simulink model "Acquisition_from_autosave"  (R2017a)
settings: Solver=VariableStepAuto  StartTime=0.0  StopTime=0.5  RelTol=1e-3
undefined symbols (not defined in the file): magnitude, Radix
libraries: simulink x34, commfilt2 x30, dspswit3 x12, dspmtrx3 x12, dspxfrm3 x3, simulink_extras x2, dspbuff3 x1
(part 1 of 4)
settings Model: Creator=Alam  LastModifiedBy=Alam
settings SolverCC: AutoInsertRateTranBlk=on
settings DataIOCC: LimitDataPoints=on  SaveOutput=off  SignalLogging=off  SaveTime=off
settings OptimizationCC: LifeSpan=inf
settings DebuggingCC: AlgebraicLoopMsg=none  SingleTaskRateTransMsg=error  AllowSymbolicDim=off  SFUnexpectedBacktrackingDiag=warning  SFNoUnconditionalDefaultTransitionDiag=warning  SFExecutionAtInitializationDiag=none
settings GRTTargetCC: TargetLangStandard=C89/C90 (ANSI)  GeneratePreprocessorConditionals=Disable all

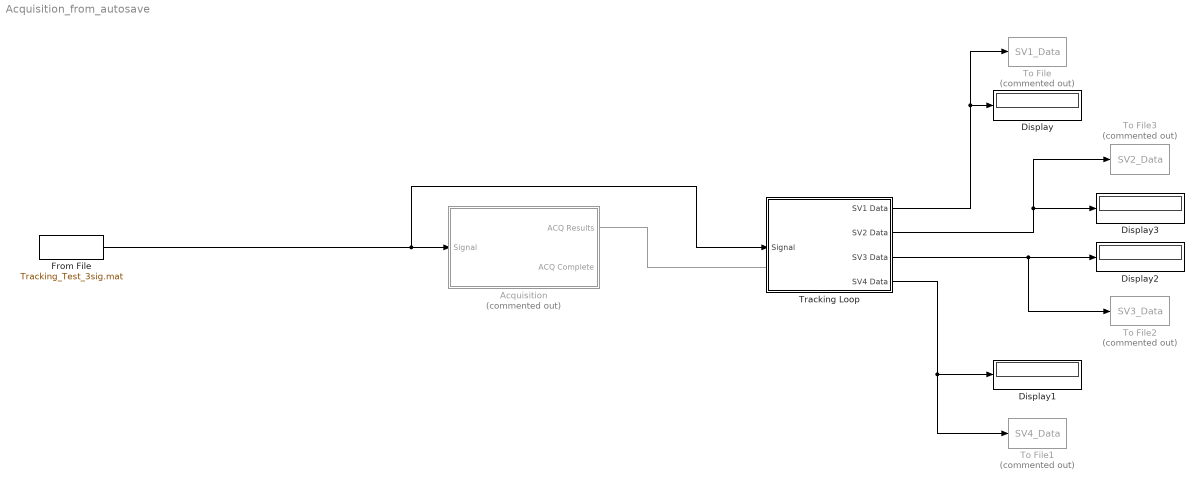
== system Acquisition_from_autosave ==
  Acquisition : Subsystem  Commented=on
  Display{,1..3} (4 alike) : Display
  From File : FromFile  FileName=Tracking_Test_3sig.mat  SampleTime=0
  To File : ToFile  Commented=on  Filename=SV1_Data  MatrixName=SV1  SampleTime=0.01
  To File1 : ToFile  Commented=on  Filename=SV4_Data  MatrixName=SV4  SampleTime=0.01
  To File2 : ToFile  Commented=on  Filename=SV3_Data  MatrixName=SV3  SampleTime=0.01
  To File3 : ToFile  Commented=on  Filename=SV2_Data  MatrixName=SV2  SampleTime=0.01
  Tracking Loop : Subsystem
      settings: MinAlgLoopOccurrences=on
  wires:
  Tracking Loop/1(SV1 Data) -> Display/1, To File/1
  Tracking Loop/4(SV4 Data) -> To File1/1, Display1/1
  Tracking Loop/3(SV3 Data) -> To File2/1, Display2/1
  Tracking Loop/2(SV2 Data) -> Display3/1, To File3/1
  Acquisition/1(ACQ Results) -> ?
  From File/1 -> Acquisition/1(Signal), Tracking Loop/1(Signal)

== system Acquisition_from_autosave/Acquisition ==
  Signal : Inport
  Array of Sattelite Info : MATLAB Function  TreatAsAtomicUnit=on  SystemSampleTime=0.021
  CA Number : dspswit3/Counter  Direction=Up  CountEvent=Rising edge  CounterSize=User defined  MaxCount=32  InitialCount=0  Output=Count  HitValue=32  ResetInput=off  SamplesPerFrame=1  Ts=1  CntDtype=double  HitDtype=Logical
  CAcode : ModelReference  ModelNameDialog=CAcode.mdl  SimulationMode=Normal  ModelReferenceVersion=1.53
  Clock : simulink_extras/Flip Flops/Clock  period=0.001
  Clock1 : simulink_extras/Flip Flops/Clock  period=0.021
  Complex to Magnitude-Angle : ComplexToMagnitudeAngle  Output=Magnitude
  Complex to Real-Imag1 : ComplexToRealImag
  "Discrete Conversion " : Subsystem
  FFT : dspxfrm3/FFT  FFTImplementation=Radix-2  CompMethod=Table lookup  TableOpt=NEW  TableOptActive=Speed  BitRevOrder=off  Normalize=off  InheritFFTLength=on  FFTLength=64  WrapInput=on  roundingMode=Floor  overflowMode=off  firstCoeffDataTypeStr=Inherit: Same word length as input  firstCoeffLastDataTypeStr=Inherit: Same word length as input  outputMin=[]  outputMax=[]
  FFT1 : dspxfrm3/FFT  FFTImplementation=Radix-2  CompMethod=Table lookup  TableOpt=NEW  TableOptActive=Speed  BitRevOrder=off  Normalize=off  InheritFFTLength=on  FFTLength=64  WrapInput=on  roundingMode=Floor  overflowMode=off  firstCoeffDataTypeStr=Inherit: Same word length as input  firstCoeffLastDataTypeStr=Inherit: Same word length as input  outputMin=[]  outputMax=[]
  Freq Step : dspswit3/Counter  Direction=Up  CountEvent=Rising edge  CounterSize=User defined  MaxCount=20  InitialCount=0  Output=Count  HitValue=32  ResetInput=off  SamplesPerFrame=1  Ts=1  CntDtype=double  HitDtype=Logical
  IFFT : dspxfrm3/IFFT  FFTImplementation=Radix-2  CompMethod=Table lookup  TableOpt=NEW  TableOptActive=Speed  BitRevOrder=off  cs_in=off  Normalize=on  InheritFFTLength=on  FFTLength=64  WrapInput=on  mode=Complex  outSamplingMode=Sample based  roundingMode=Floor  overflowMode=off  firstCoeffDataTypeStr=Inherit: Same word length as input  firstCoeffLastDataTypeStr=Inherit: Same word length as input  outputMin=[]  outputMax=[]
      settings: SourceProductName=DSP System Toolbox
  Math Function : Math  Operator=conj  SaturateOnIntegerOverflow=on
  Non-Return to Zero : Subsystem
  Oscillator : ModelReference  ModelNameDialog=Local_Oscillator.slx  SimulationMode=Normal  ModelReferenceVersion=1.39
  Product{,1..3} (4 alike) : Product
  RT : RateTransition  OutPortSampleTime=0.021
  Rate Transition : RateTransition
  Real-Imag to Complex : RealImagToComplex
  Reshape : Reshape  OutputDimensionality=Column vector (2-D)
  Search Correlation Data : Subsystem
  ACQ Results : Outport
  ACQ Complete : Outport  Port=2
  wires:
  Array of Sattelite Info/1(Visible_Satellites) -> ACQ Results/1
  Array of Sattelite Info/2(Complete) -> ACQ Complete/1
  FFT1/1 -> Math Function/1
  CAcode/1 -> Reshape/1
  Product1/1 -> Real-Imag to Complex/2
  Oscillator/1 -> Complex to Real-Imag1/1
  IFFT/1 -> Complex to Magnitude-Angle/1
  Rate Transition/1 -> Oscillator/1
  Complex to Real-Imag1/1 -> Product/2
  Math Function/1 -> Product2/2
  Complex to Magnitude-Angle/1 -> Product3/1, Product3/2
  Clock1/1 -> CA Number/1
  Product3/1 -> Search Correlation Data/1(In1)
  Search Correlation Data/1(Out1) -> RT/1
  Clock/1 -> Freq Step/1
  Freq Step/1 -> Rate Transition/1, Search Correlation Data/3(In3)
  "Discrete Conversion "/1(Out1) -> FFT/1
  FFT/1 -> Product2/1
  Reshape/1 -> Non-Return to Zero/1(In1)
  Real-Imag to Complex/1 -> "Discrete Conversion "/1(In1)
  Non-Return to Zero/1(Out1) -> FFT1/1
  CA Number/1 -> Search Correlation Data/2(In2), CAcode/1
  Product2/1 -> IFFT/1
  Product/1 -> Real-Imag to Complex/1
  Signal/1 -> Product/1, Product1/1
  Complex to Real-Imag1/2 -> Product1/2
  RT/1 -> Array of Sattelite Info/1(input_vector)

== system Acquisition_from_autosave/Tracking Loop ==
  Signal : Inport
  MATLAB Function : MATLAB Function  TreatAsAtomicUnit=on
  SV Parameter Fetch : Subsystem
  Scope : Scope  NumInputPorts=4
  Scope1 : Scope  NumInputPorts=4
  Sign{,1..3} (4 alike) : Signum
  Tracking Loops : Subsystem
  SV1 Data : Outport
  SV2 Data : Outport  Port=2
  SV3 Data : Outport  Port=3
  SV4 Data : Outport  Port=4
  wires:
  MATLAB Function/1(y) -> SV Parameter Fetch/1(ACQ results)
  SV Parameter Fetch/1(PRN_SV_1) -> Tracking Loops/2(In2)
  SV Parameter Fetch/2(Freq_SV_1) -> Tracking Loops/3(In3)
  SV Parameter Fetch/3(CodePhase_SV_1) -> Tracking Loops/4(In4)
  SV Parameter Fetch/4(PRN_SV_2) -> Tracking Loops/5(In5)
  SV Parameter Fetch/5(Freq_SV_2) -> Tracking Loops/6(In6)
  SV Parameter Fetch/6(CodePhase_SV_2) -> Tracking Loops/7(In7)
  SV Parameter Fetch/7(PRN_SV_3) -> Tracking Loops/8(In8)
  SV Parameter Fetch/8(Freq_SV_3) -> Tracking Loops/9(In9)
  SV Parameter Fetch/9(CodePhase_SV_3) -> Tracking Loops/10(In10)
  SV Parameter Fetch/10(PRN_SV_4) -> Tracking Loops/11(In11)
  SV Parameter Fetch/11(Freq_SV_4) -> Tracking Loops/12(In12)
  SV Parameter Fetch/12(CodePhase_SV_4) -> Tracking Loops/13(In13)
  Signal/1 -> Tracking Loops/1(In1)
  Tracking Loops/1(SV1 Data) -> Sign/1, Scope1/1, SV1 Data/1
  Tracking Loops/2(SV2 Data) -> Scope1/2, SV2 Data/1, Sign1/1
  Tracking Loops/3(SV3 Data) -> Sign3/1, Scope1/3, SV3 Data/1
  Tracking Loops/4(SV4 Data) -> Scope1/4, Sign2/1, SV4 Data/1
  Sign/1 -> Scope/1
  Sign1/1 -> Scope/2
  Sign2/1 -> Scope/4
  Sign3/1 -> Scope/3

== system Acquisition_from_autosave/Acquisition/Discrete Conversion  ==
  In1 : Inport
  Delay Line : dspbuff3/Delay Line  siz=32768  ic=0  directfeed=off  enable_output=off  hold_output=off  OutputFrames=off
      settings: SourceProductName=DSP System Toolbox  SourceProductBaseCode=DS
  Zero-Order Hold : ZeroOrderHold  SampleTime=3.05175781e-8
  Out1 : Outport  SampleTime=0.001
  wires:
  Delay Line/1 -> Out1/1
  Zero-Order Hold/1 -> Delay Line/1
  In1/1 -> Zero-Order Hold/1

== system Acquisition_from_autosave/Acquisition/Non-Return to Zero ==
  In1 : Inport
  Constant2 : Constant  Value=2
  Constant6 : Constant  Value=-1
  Product4 : Product
  Sum : Sum  Inputs=|++
  Out1 : Outport
  wires:
  Sum/1 -> Out1/1
  Constant2/1 -> Product4/1
  Product4/1 -> Sum/1
  In1/1 -> Product4/2
  Constant6/1 -> Sum/2

== system Acquisition_from_autosave/Acquisition/Search Correlation Data ==
  In1 : Inport  PortDimensions=[32768 1]  SampleTime=0.001
  In2 : Inport  Port=2  SampleTime=0.001
  In3 : Inport  Port=3  SampleTime=0.001
  MATLAB Function : MATLAB Function  TreatAsAtomicUnit=on  SystemSampleTime=0.001
  Out1 : Outport
  wires:
  MATLAB Function/1(Sat) -> Out1/1
  In3/1 -> MATLAB Function/3(freq_step)
  In1/1 -> MATLAB Function/1(vector)
  In2/1 -> MATLAB Function/2(PRN)

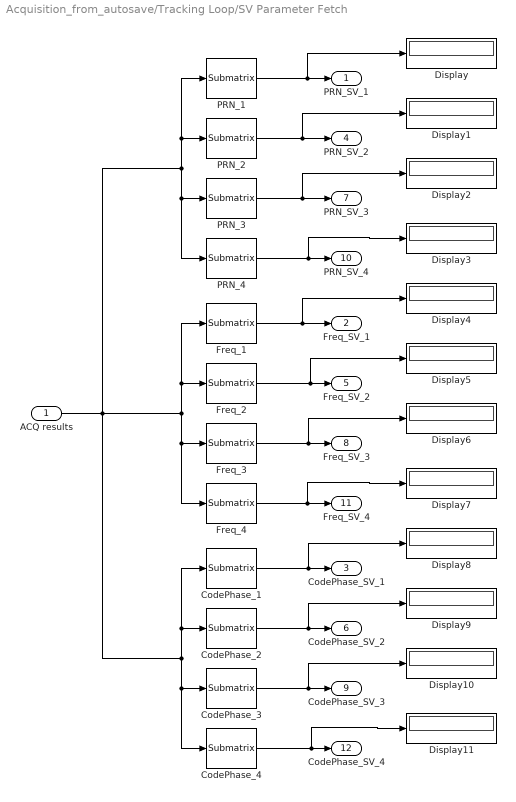
== system Acquisition_from_autosave/Tracking Loop/SV Parameter Fetch ==
  ACQ results : Inport
  CodePhase_1 : dspmtrx3/Submatrix  RowSpan=One row  RowStartMode=Index  RowStartIndex=1  RowEndMode=Last  RowEndIndex=1  ColSpan=One column  ColStartMode=Index  ColStartIndex=4  ColEndMode=Last  ColEndIndex=1
  CodePhase_2 : dspmtrx3/Submatrix  RowSpan=One row  RowStartMode=Index  RowStartIndex=2  RowEndMode=Last  RowEndIndex=1  ColSpan=One column  ColStartMode=Index  ColStartIndex=4  ColEndMode=Last  ColEndIndex=1
  CodePhase_3 : dspmtrx3/Submatrix  RowSpan=One row  RowStartMode=Index  RowStartIndex=3  RowEndMode=Last  RowEndIndex=1  ColSpan=One column  ColStartMode=Index  ColStartIndex=4  ColEndMode=Last  ColEndIndex=1
  CodePhase_4 : dspmtrx3/Submatrix  RowSpan=One row  RowStartMode=Index  RowStartIndex=4  RowEndMode=Last  RowEndIndex=1  ColSpan=One column  ColStartMode=Index  ColStartIndex=4  ColEndMode=Last  ColEndIndex=1
  Display{,1..11} (12 alike) : Display
  Freq_1 : dspmtrx3/Submatrix  RowSpan=One row  RowStartMode=Index  RowStartIndex=1  RowEndMode=Last  RowEndIndex=1  ColSpan=One column  ColStartMode=Index  ColStartIndex=3  ColEndMode=Last  ColEndIndex=1
  Freq_2 : dspmtrx3/Submatrix  RowSpan=One row  RowStartMode=Index  RowStartIndex=2  RowEndMode=Last  RowEndIndex=1  ColSpan=One column  ColStartMode=Index  ColStartIndex=3  ColEndMode=Last  ColEndIndex=1
  Freq_3 : dspmtrx3/Submatrix  RowSpan=One row  RowStartMode=Index  RowStartIndex=3  RowEndMode=Last  RowEndIndex=1  ColSpan=One column  ColStartMode=Index  ColStartIndex=3  ColEndMode=Last  ColEndIndex=1
  Freq_4 : dspmtrx3/Submatrix  RowSpan=One row  RowStartMode=Index  RowStartIndex=4  RowEndMode=Last  RowEndIndex=1  ColSpan=One column  ColStartMode=Index  ColStartIndex=3  ColEndMode=Last  ColEndIndex=1
  PRN_1 : dspmtrx3/Submatrix  RowSpan=One row  RowStartMode=Index  RowStartIndex=1  RowEndMode=Last  RowEndIndex=1  ColSpan=One column  ColStartMode=Index  ColStartIndex=2  ColEndMode=Last  ColEndIndex=1
  PRN_2 : dspmtrx3/Submatrix  RowSpan=One row  RowStartMode=Index  RowStartIndex=2  RowEndMode=Last  RowEndIndex=1  ColSpan=One column  ColStartMode=Index  ColStartIndex=2  ColEndMode=Last  ColEndIndex=1
  PRN_3 : dspmtrx3/Submatrix  RowSpan=One row  RowStartMode=Index  RowStartIndex=3  RowEndMode=Last  RowEndIndex=1  ColSpan=One column  ColStartMode=Index  ColStartIndex=2  ColEndMode=Last  ColEndIndex=1
  PRN_4 : dspmtrx3/Submatrix  RowSpan=One row  RowStartMode=Index  RowStartIndex=4  RowEndMode=Last  RowEndIndex=1  ColSpan=One column  ColStartMode=Index  ColStartIndex=2  ColEndMode=Last  ColEndIndex=1
  PRN_SV_1 : Outport
  Freq_SV_1 : Outport  Port=2
  CodePhase_SV_1 : Outport  Port=3
  PRN_SV_2 : Outport  Port=4
  Freq_SV_2 : Outport  Port=5
  CodePhase_SV_2 : Outport  Port=6
  PRN_SV_3 : Outport  Port=7
  Freq_SV_3 : Outport  Port=8
  CodePhase_SV_3 : Outport  Port=9
  PRN_SV_4 : Outport  Port=10
  Freq_SV_4 : Outport  Port=11
  CodePhase_SV_4 : Outport  Port=12
  wires:
  ACQ results/1 -> CodePhase_4/1, CodePhase_3/1, CodePhase_2/1, CodePhase_1/1, Freq_4/1, Freq_3/1, Freq_2/1, Freq_1/1, PRN_4/1, PRN_3/1, PRN_2/1, PRN_1/1
  PRN_1/1 -> Display/1, PRN_SV_1/1
  PRN_2/1 -> Display1/1, PRN_SV_2/1
  PRN_3/1 -> Display2/1, PRN_SV_3/1
  PRN_4/1 -> Display3/1, PRN_SV_4/1
  Freq_1/1 -> Display4/1, Freq_SV_1/1
  Freq_2/1 -> Display5/1, Freq_SV_2/1
  Freq_3/1 -> Display6/1, Freq_SV_3/1
  Freq_4/1 -> Display7/1, Freq_SV_4/1
  CodePhase_1/1 -> Display8/1, CodePhase_SV_1/1
  CodePhase_2/1 -> Display9/1, CodePhase_SV_2/1
  CodePhase_3/1 -> Display10/1, CodePhase_SV_3/1
  CodePhase_4/1 -> Display11/1, CodePhase_SV_4/1

== system Acquisition_from_autosave/Tracking Loop/Tracking Loops ==
  In1 : Inport
  In2 : Inport  Port=2
  In3 : Inport  Port=3
  In4 : Inport  Port=4
  In5 : Inport  Port=5
  In6 : Inport  Port=6
  In7 : Inport  Port=7
  In8 : Inport  Port=8
  In9 : Inport  Port=9
  In10 : Inport  Port=10
  In11 : Inport  Port=11
  In12 : Inport  Port=12
  In13 : Inport  Port=13
  Carrier Error : Scope  NumInputPorts=4
  Code Phase Error : Scope  NumInputPorts=4
  From File : FromFile  FileName=Tracking_Test_3sig_1.mat  SampleTime=0
  From File1 : FromFile  FileName=Tracking_Test_3sig_2.mat  SampleTime=0
  From File2 : FromFile  FileName=Tracking_Test_3sig_3.mat  SampleTime=0
  From File3 : FromFile  FileName=Tracking_Test_3sig_4.mat  SampleTime=0
  Sum : Sum  Inputs=|++++|
  Tracking Loop1 : Subsystem  Commented=on  TreatAsAtomicUnit=on
      settings: MinAlgLoopOccurrences=on
  Tracking Loop2 : Subsystem  Commented=on  TreatAsAtomicUnit=on
      settings: MinAlgLoopOccurrences=on
  Tracking Loop3 : Subsystem  TreatAsAtomicUnit=on
      settings: MinAlgLoopOccurrences=on
  Tracking Loop4 : Subsystem  TreatAsAtomicUnit=on
      settings: MinAlgLoopOccurrences=on
  Tracking Loop5 : Subsystem  TreatAsAtomicUnit=on
      settings: MinAlgLoopOccurrences=on
  SV1 Data : Outport
  SV2 Data : Outport  Port=2
  SV3 Data : Outport  Port=3
  SV4 Data : Outport  Port=4
  wires:
  Sum/1 -> Tracking Loop1/1(Input Signal), Tracking Loop5/1(Input Signal), Tracking Loop4/1(Input Signal), Tracking Loop3/1(Input Signal)
  Tracking Loop1/1(Data) -> SV1 Data/1
  Tracking Loop4/1(Data) -> SV4 Data/1
  Tracking Loop3/1(Data) -> SV3 Data/1
  In12/1 -> Tracking Loop4/3(Frequency)
  In3/1 -> Tracking Loop1/3(Frequency)
  In4/1 -> Tracking Loop1/4(Code Phase1)
  In6/1 -> Tracking Loop5/3(Frequency)
  In13/1 -> Tracking Loop4/4(Code Phase1)
  In9/1 -> Tracking Loop3/3(Frequency)
  In8/1 -> Tracking Loop3/2(PRN)
  In11/1 -> Tracking Loop4/2(PRN)
  In5/1 -> Tracking Loop5/2(PRN)
  In10/1 -> Tracking Loop3/4(Code Phase1)
  In2/1 -> Tracking Loop1/2(PRN)
  In7/1 -> Tracking Loop5/4(Code Phase1)
  Tracking Loop5/1(Data) -> SV2 Data/1
  ? -> Carrier Error/1
  Tracking Loop5/2(filter error) -> Carrier Error/2
  Tracking Loop3/2(filter error) -> Carrier Error/3
  Tracking Loop4/2(filter error) -> Carrier Error/4
  Tracking Loop3/3(code_phase_error) -> Code Phase Error/3
  Tracking Loop4/3(code_phase_error) -> Code Phase Error/4
  ? -> Code Phase Error/1
  Tracking Loop5/3(code_phase_error) -> Code Phase Error/2
  From File/1 -> Sum/1
  From File1/1 -> Sum/2
  From File2/1 -> Sum/3
  From File3/1 -> Sum/4

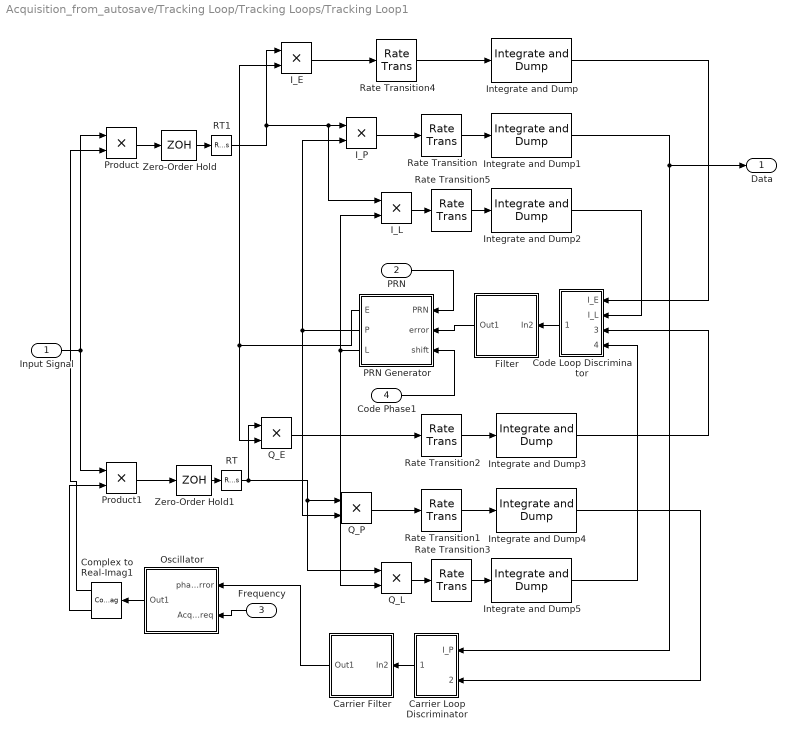
== system Acquisition_from_autosave/Tracking Loop/Tracking Loops/Tracking Loop1 ==
  Input Signal : Inport
  PRN : Inport  Port=2
  Frequency : Inport  Port=3
  Code Phase1 : Inport  Port=4
  Carrier Filter : Subsystem
  "Carrier Loop Discriminator " : Subsystem
  Code Loop Discriminator : Subsystem
  Complex to Real-Imag1 : ComplexToRealImag
  Filter : Subsystem
  I_E : Product
  I_L : Product
  "I_P " : Product
  Integrate and Dump{,1..5} (6 alike) : commfilt2/Integrate and Dump  obssamples=32768  offsetsamples=0  nodump=off  roundingMode=Floor  overflowMode=off  outputDataTypeStr=Inherit: Same as accumulator  outputLastDataTypeStr=Inherit: Same as accumulator
      settings: SourceProductName=Communications System Toolbox
  Oscillator : Subsystem
  "PRN Generator " : Subsystem
  Product : Product
  Product1 : Product
  Q_E : Product
  Q_L : Product
  Q_P : Product
  RT : RateTransition
  RT1 : RateTransition
  Rate Transition{,1..5} (6 alike) : RateTransition  OutPortSampleTime=3.0517578125e-8
  Zero-Order Hold : ZeroOrderHold  SampleTime=3.0517578125e-8
  Zero-Order Hold1 : ZeroOrderHold  SampleTime=3.0517578125e-8
  Data : Outport
  wires:
  I_L/1 -> Rate Transition5/1
  "PRN Generator "/3(L) -> Q_L/2, I_L/2
  Q_E/1 -> Rate Transition2/1
  Q_L/1 -> Rate Transition3/1
  "PRN Generator "/2(P) -> Q_P/2, "I_P "/2
  Q_P/1 -> Rate Transition1/1
  "I_P "/1 -> Rate Transition/1
  "Carrier Loop Discriminator "/1(theta) -> Carrier Filter/1(In2)
  Rate Transition/1 -> Integrate and Dump1/1
  Rate Transition4/1 -> Integrate and Dump/1
  RT/1 -> Q_L/1, Q_P/1, Q_E/1
  Code Phase1/1 -> "PRN Generator "/3(shift)
  Product/1 -> Zero-Order Hold/1
  PRN/1 -> "PRN Generator "/1(PRN)
  Complex to Real-Imag1/2 -> Product1/2
  Input Signal/1 -> Product1/1, Product/1
  Complex to Real-Imag1/1 -> Product/2
  I_E/1 -> Rate Transition4/1
  Integrate and Dump/1 -> Code Loop Discriminator/1(I_E)
  Integrate and Dump5/1 -> Code Loop Discriminator/4(Q_L)
  Integrate and Dump3/1 -> Code Loop Discriminator/3(Q_E)
  "PRN Generator "/1(E) -> I_E/2, Q_E/2
  Integrate and Dump2/1 -> Code Loop Discriminator/2(I_L)
  Rate Transition1/1 -> Integrate and Dump4/1
  Rate Transition3/1 -> Integrate and Dump5/1
  Rate Transition2/1 -> Integrate and Dump3/1
  Rate Transition5/1 -> Integrate and Dump2/1
  Frequency/1 -> Oscillator/2(Acq Freq)
  Product1/1 -> Zero-Order Hold1/1
  Zero-Order Hold/1 -> RT1/1
  RT1/1 -> I_E/1, I_L/1, "I_P "/1
  Zero-Order Hold1/1 -> RT/1
  Oscillator/1(Out1) -> Complex to Real-Imag1/1
  Carrier Filter/1(Out1) -> Oscillator/1(phase error)
  Integrate and Dump4/1 -> "Carrier Loop Discriminator "/2(Q_P)
  Integrate and Dump1/1 -> "Carrier Loop Discriminator "/1(I_P), Data/1
  Filter/1(Out1) -> "PRN Generator "/2(error)
  Code Loop Discriminator/1(error) -> Filter/1(In2)

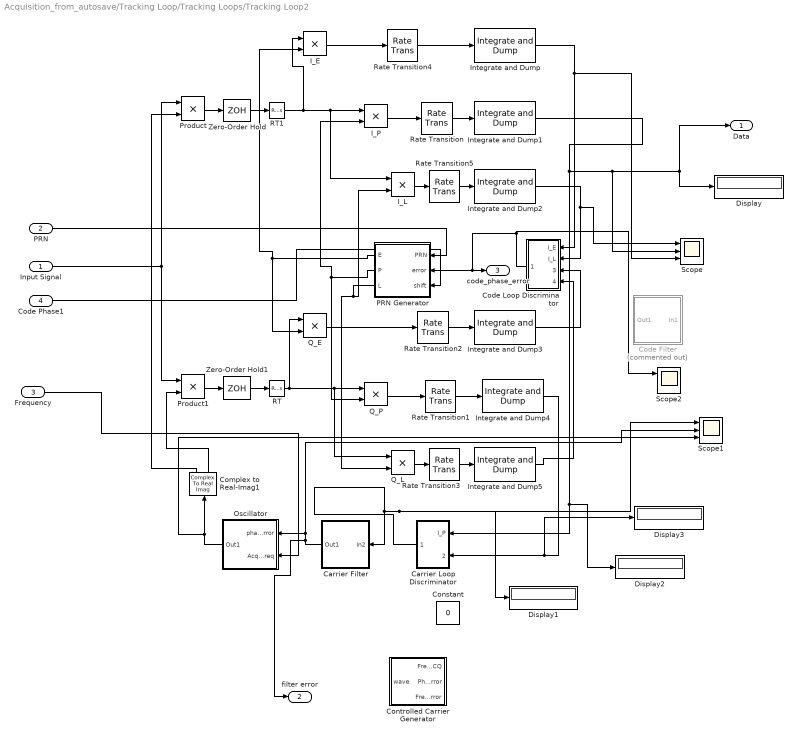
== system Acquisition_from_autosave/Tracking Loop/Tracking Loops/Tracking Loop2 ==
  Input Signal : Inport
  PRN : Inport  Port=2
  Frequency : Inport  Port=3
  Code Phase1 : Inport  Port=4
  Carrier Filter : Subsystem
  "Carrier Loop Discriminator " : Subsystem
  Code Filter : Subsystem  Commented=on
  Code Loop Discriminator : Subsystem
  Complex to Real-Imag1 : ComplexToRealImag
  Constant : Constant  Value=0  SampleTime=0.001
  Controlled Carrier Generator : Subsystem
  Display{,1..3} (4 alike) : Display
  I_E : Product
  I_L : Product
  "I_P " : Product
  Integrate and Dump{,1..5} (6 alike) : commfilt2/Integrate and Dump  obssamples=32768  offsetsamples=0  nodump=off  roundingMode=Floor  overflowMode=off  outputDataTypeStr=Inherit: Same as accumulator  outputLastDataTypeStr=Inherit: Same as accumulator
      settings: SourceProductName=Communications System Toolbox
  Oscillator : Subsystem
  "PRN Generator " : Subsystem
  Product : Product
  Product1 : Product
  Q_E : Product
  Q_L : Product
  Q_P : Product
  RT : RateTransition
  RT1 : RateTransition
  Rate Transition{,1..5} (6 alike) : RateTransition  OutPortSampleTime=3.0517578125e-8
  Scope : Scope  NumInputPorts=3
  Scope1 : Scope  NumInputPorts=3
  Scope2 : Scope  NumInputPorts=3
  Zero-Order Hold : ZeroOrderHold  SampleTime=3.0517578125e-8
  Zero-Order Hold1 : ZeroOrderHold  SampleTime=3.0517578125e-8
  Data : Outport
  filter error : Outport  Port=2
  code_phase_error : Outport  Port=3
  wires:
  I_L/1 -> Rate Transition5/1
  "PRN Generator "/3(L) -> Q_L/2, I_L/2
  Q_E/1 -> Rate Transition2/1
  Q_L/1 -> Rate Transition3/1
  "PRN Generator "/2(P) -> "I_P "/2, Q_P/2
  Q_P/1 -> Rate Transition1/1
  "I_P "/1 -> Rate Transition/1
  "Carrier Loop Discriminator "/1(theta) -> Carrier Filter/1(In2), Scope1/1, Display1/1
  Rate Transition/1 -> Integrate and Dump1/1
  Rate Transition4/1 -> Integrate and Dump/1
  RT/1 -> Q_L/1, Q_P/1, Q_E/1
  Code Phase1/1 -> "PRN Generator "/3(shift)
  Product/1 -> Zero-Order Hold/1
  PRN/1 -> "PRN Generator "/1(PRN)
  Complex to Real-Imag1/2 -> Product1/2
  Input Signal/1 -> Product1/1, Product/1
  Complex to Real-Imag1/1 -> Product/2
  I_E/1 -> Rate Transition4/1
  Integrate and Dump/1 -> Scope/3, Code Loop Discriminator/1(I_E)
  Integrate and Dump5/1 -> Code Loop Discriminator/4(Q_L)
  Integrate and Dump3/1 -> Code Loop Discriminator/3(Q_E)
  "PRN Generator "/1(E) -> I_E/2, Q_E/2
  Integrate and Dump4/1 -> Display3/1, "Carrier Loop Discriminator "/2(Q_P)
  Integrate and Dump2/1 -> Scope/1, Code Loop Discriminator/2(I_L)
  Rate Transition1/1 -> Integrate and Dump4/1
  Rate Transition3/1 -> Integrate and Dump5/1
  Rate Transition2/1 -> Integrate and Dump3/1
  Rate Transition5/1 -> Integrate and Dump2/1
  Frequency/1 -> Oscillator/2(Acq Freq)
  Product1/1 -> Zero-Order Hold1/1
  Zero-Order Hold/1 -> RT1/1
  RT1/1 -> I_E/1, I_L/1, "I_P "/1
  Integrate and Dump1/1 -> Scope/2, Display/1, Data/1, Display2/1, "Carrier Loop Discriminator "/1(I_P)
  Zero-Order Hold1/1 -> RT/1
  Oscillator/1(Out1) -> Scope1/3, Complex to Real-Imag1/1
  Carrier Filter/1(Out1) -> filter error/1, Oscillator/1(phase error), Scope1/2
  Code Loop Discriminator/1(error) -> "PRN Generator "/2(error), code_phase_error/1, Scope2/1

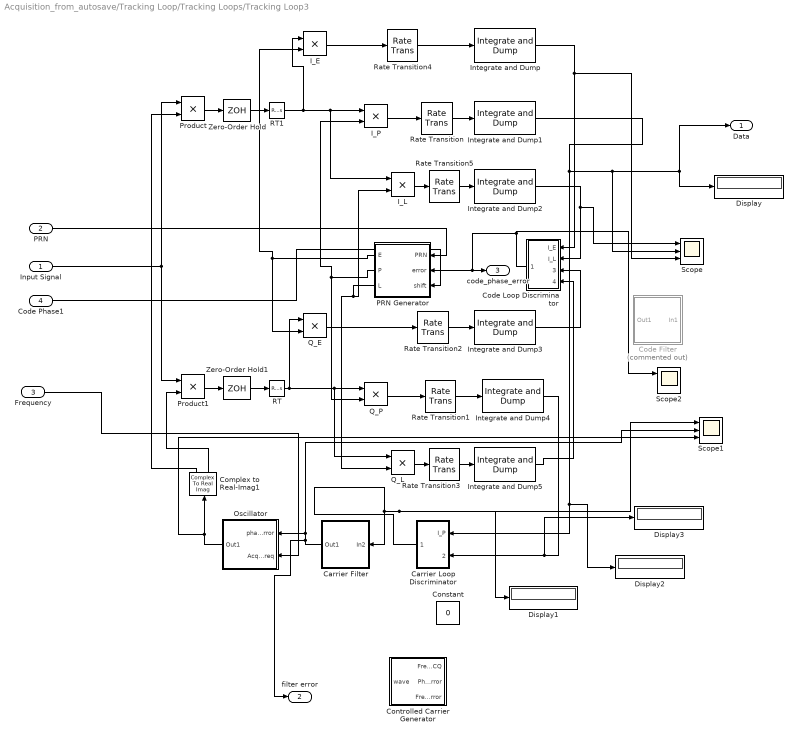
== system Acquisition_from_autosave/Tracking Loop/Tracking Loops/Tracking Loop3 ==
  Input Signal : Inport
  PRN : Inport  Port=2
  Frequency : Inport  Port=3
  Code Phase1 : Inport  Port=4
  Carrier Filter : Subsystem
  "Carrier Loop Discriminator " : Subsystem
  Code Filter : Subsystem  Commented=on
  Code Loop Discriminator : Subsystem
  Complex to Real-Imag1 : ComplexToRealImag
  Constant : Constant  Value=0  SampleTime=0.001
  Controlled Carrier Generator : Subsystem
  Display{,1..3} (4 alike) : Display
  I_E : Product
  I_L : Product
  "I_P " : Product
  Integrate and Dump{,1..5} (6 alike) : commfilt2/Integrate and Dump  obssamples=32768  offsetsamples=0  nodump=off  roundingMode=Floor  overflowMode=off  outputDataTypeStr=Inherit: Same as accumulator  outputLastDataTypeStr=Inherit: Same as accumulator
      settings: SourceProductName=Communications System Toolbox
  Oscillator : Subsystem
  "PRN Generator " : Subsystem
  Product : Product
  Product1 : Product
  Q_E : Product
  Q_L : Product
  Q_P : Product
  RT : RateTransition
  RT1 : RateTransition
  Rate Transition{,1..5} (6 alike) : RateTransition  OutPortSampleTime=3.0517578125e-8
  Scope : Scope  NumInputPorts=3
  Scope1 : Scope  NumInputPorts=3
  Scope2 : Scope  NumInputPorts=3
  Zero-Order Hold : ZeroOrderHold  SampleTime=3.0517578125e-8
  Zero-Order Hold1 : ZeroOrderHold  SampleTime=3.0517578125e-8
  Data : Outport
  filter error : Outport  Port=2
  code_phase_error : Outport  Port=3
  wires:
  I_L/1 -> Rate Transition5/1
  "PRN Generator "/3(L) -> Q_L/2, I_L/2
  Q_E/1 -> Rate Transition2/1
  Q_L/1 -> Rate Transition3/1
  "PRN Generator "/2(P) -> "I_P "/2, Q_P/2
  Q_P/1 -> Rate Transition1/1
  "I_P "/1 -> Rate Transition/1
  "Carrier Loop Discriminator "/1(theta) -> Carrier Filter/1(In2), Scope1/1, Display1/1
  Rate Transition/1 -> Integrate and Dump1/1
  Rate Transition4/1 -> Integrate and Dump/1
  RT/1 -> Q_L/1, Q_P/1, Q_E/1
  Code Phase1/1 -> "PRN Generator "/3(shift)
  Product/1 -> Zero-Order Hold/1
  PRN/1 -> "PRN Generator "/1(PRN)
  Complex to Real-Imag1/2 -> Product1/2
  Input Signal/1 -> Product1/1, Product/1
  Complex to Real-Imag1/1 -> Product/2
  I_E/1 -> Rate Transition4/1
  Integrate and Dump/1 -> Scope/3, Code Loop Discriminator/1(I_E)
  Integrate and Dump5/1 -> Code Loop Discriminator/4(Q_L)
  Integrate and Dump3/1 -> Code Loop Discriminator/3(Q_E)
  "PRN Generator "/1(E) -> I_E/2, Q_E/2
  Integrate and Dump2/1 -> Scope/1, Code Loop Discriminator/2(I_L)
  Rate Transition1/1 -> Integrate and Dump4/1
  Rate Transition3/1 -> Integrate and Dump5/1
  Rate Transition2/1 -> Integrate and Dump3/1
  Rate Transition5/1 -> Integrate and Dump2/1
  Frequency/1 -> Oscillator/2(Acq Freq)
  Product1/1 -> Zero-Order Hold1/1
  Zero-Order Hold/1 -> RT1/1
  RT1/1 -> I_E/1, I_L/1, "I_P "/1
  Zero-Order Hold1/1 -> RT/1
  Oscillator/1(Out1) -> Scope1/3, Complex to Real-Imag1/1
  Carrier Filter/1(Out1) -> filter error/1, Oscillator/1(phase error), Scope1/2
  Code Loop Discriminator/1(error) -> "PRN Generator "/2(error), code_phase_error/1, Scope2/1
  Integrate and Dump4/1 -> "Carrier Loop Discriminator "/2(Q_P), Display3/1
  Integrate and Dump1/1 -> Scope/2, Display/1, Data/1, "Carrier Loop Discriminator "/1(I_P), Display2/1

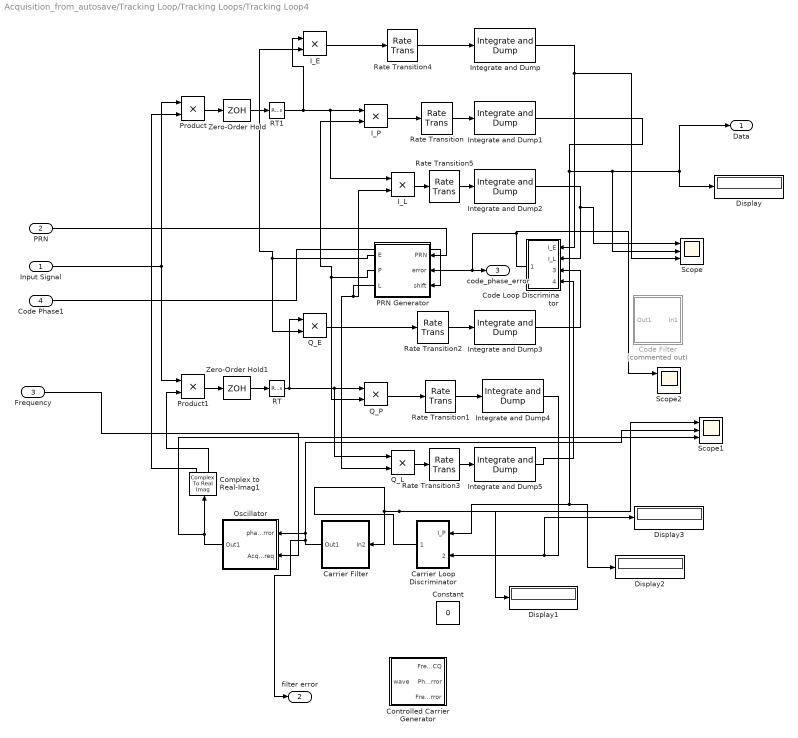
== system Acquisition_from_autosave/Tracking Loop/Tracking Loops/Tracking Loop4 ==
  Input Signal : Inport
  PRN : Inport  Port=2
  Frequency : Inport  Port=3
  Code Phase1 : Inport  Port=4
  Carrier Filter : Subsystem
  "Carrier Loop Discriminator " : Subsystem
  Code Filter : Subsystem  Commented=on
  Code Loop Discriminator : Subsystem
  Complex to Real-Imag1 : ComplexToRealImag
  Constant : Constant  Value=0  SampleTime=0.001
  Controlled Carrier Generator : Subsystem
  Display{,1..3} (4 alike) : Display
  I_E : Product
  I_L : Product
  "I_P " : Product
  Integrate and Dump{,1..5} (6 alike) : commfilt2/Integrate and Dump  obssamples=32768  offsetsamples=0  nodump=off  roundingMode=Floor  overflowMode=off  outputDataTypeStr=Inherit: Same as accumulator  outputLastDataTypeStr=Inherit: Same as accumulator
      settings: SourceProductName=Communications System Toolbox
  Oscillator : Subsystem
  "PRN Generator " : Subsystem
  Product : Product
  Product1 : Product
  Q_E : Product
  Q_L : Product
  Q_P : Product
  RT : RateTransition
  RT1 : RateTransition
  Rate Transition{,1..5} (6 alike) : RateTransition  OutPortSampleTime=3.0517578125e-8
  Scope : Scope  NumInputPorts=3
  Scope1 : Scope  NumInputPorts=3
  Scope2 : Scope  NumInputPorts=3
  Zero-Order Hold : ZeroOrderHold  SampleTime=3.0517578125e-8
  Zero-Order Hold1 : ZeroOrderHold  SampleTime=3.0517578125e-8
  Data : Outport
  filter error : Outport  Port=2
  code_phase_error : Outport  Port=3
  wires:
  I_L/1 -> Rate Transition5/1
  "PRN Generator "/3(L) -> Q_L/2, I_L/2
  Q_E/1 -> Rate Transition2/1
  Q_L/1 -> Rate Transition3/1
  "PRN Generator "/2(P) -> "I_P "/2, Q_P/2
  Q_P/1 -> Rate Transition1/1
  "I_P "/1 -> Rate Transition/1
  "Carrier Loop Discriminator "/1(theta) -> Carrier Filter/1(In2), Scope1/1, Display1/1
  Rate Transition/1 -> Integrate and Dump1/1
  Rate Transition4/1 -> Integrate and Dump/1
  RT/1 -> Q_L/1, Q_P/1, Q_E/1
  Code Phase1/1 -> "PRN Generator "/3(shift)
  Product/1 -> Zero-Order Hold/1
  PRN/1 -> "PRN Generator "/1(PRN)
  Complex to Real-Imag1/2 -> Product1/2
  Input Signal/1 -> Product1/1, Product/1
  Complex to Real-Imag1/1 -> Product/2
  I_E/1 -> Rate Transition4/1
  Integrate and Dump/1 -> Scope/3, Code Loop Discriminator/1(I_E)
  Integrate and Dump5/1 -> Code Loop Discriminator/4(Q_L)
  Integrate and Dump3/1 -> Code Loop Discriminator/3(Q_E)
  "PRN Generator "/1(E) -> I_E/2, Q_E/2
  Integrate and Dump2/1 -> Scope/1, Code Loop Discriminator/2(I_L)
  Rate Transition1/1 -> Integrate and Dump4/1
  Rate Transition3/1 -> Integrate and Dump5/1
  Rate Transition2/1 -> Integrate and Dump3/1
  Rate Transition5/1 -> Integrate and Dump2/1
  Frequency/1 -> Oscillator/2(Acq Freq)
  Product1/1 -> Zero-Order Hold1/1
  Zero-Order Hold/1 -> RT1/1
  RT1/1 -> I_E/1, I_L/1, "I_P "/1
  Zero-Order Hold1/1 -> RT/1
  Oscillator/1(Out1) -> Scope1/3, Complex to Real-Imag1/1
  Carrier Filter/1(Out1) -> filter error/1, Oscillator/1(phase error), Scope1/2
  Code Loop Discriminator/1(error) -> "PRN Generator "/2(error), code_phase_error/1, Scope2/1
  Integrate and Dump4/1 -> "Carrier Loop Discriminator "/2(Q_P), Display3/1
  Integrate and Dump1/1 -> Scope/2, Display/1, Data/1, "Carrier Loop Discriminator "/1(I_P), Display2/1

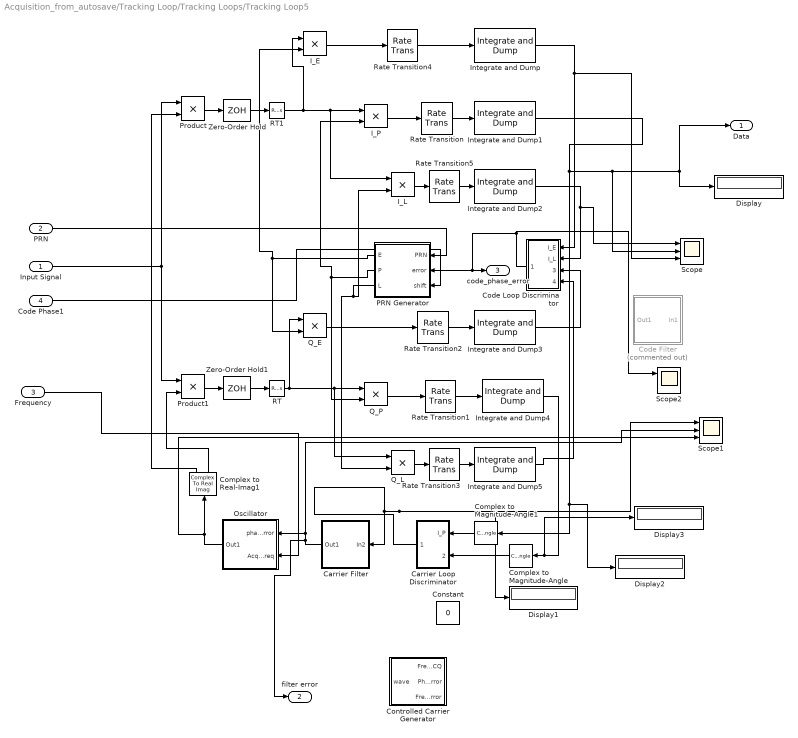
== system Acquisition_from_autosave/Tracking Loop/Tracking Loops/Tracking Loop5 ==
  Input Signal : Inport
  PRN : Inport  Port=2
  Frequency : Inport  Port=3
  Code Phase1 : Inport  Port=4
  Carrier Filter : Subsystem
  "Carrier Loop Discriminator " : Subsystem
  Code Filter : Subsystem  Commented=on
  Code Loop Discriminator : Subsystem
  Complex to Magnitude-Angle : ComplexToMagnitudeAngle  Output=Magnitude
  Complex to Magnitude-Angle1 : ComplexToMagnitudeAngle  Output=Magnitude
  Complex to Real-Imag1 : ComplexToRealImag
  Constant : Constant  Value=0  SampleTime=0.001
  Controlled Carrier Generator : Subsystem
  Display{,1..3} (4 alike) : Display
  I_E : Product
  I_L : Product
  "I_P " : Product
  Integrate and Dump{,1..5} (6 alike) : commfilt2/Integrate and Dump  obssamples=32768  offsetsamples=0  nodump=off  roundingMode=Floor  overflowMode=off  outputDataTypeStr=Inherit: Same as accumulator  outputLastDataTypeStr=Inherit: Same as accumulator
      settings: SourceProductName=Communications System Toolbox
  Oscillator : Subsystem
  "PRN Generator " : Subsystem
  Product : Product
  Product1 : Product
  Q_E : Product
  Q_L : Product
  Q_P : Product
  RT : RateTransition
  RT1 : RateTransition
  Rate Transition{,1..5} (6 alike) : RateTransition  OutPortSampleTime=3.0517578125e-8
  Scope : Scope  NumInputPorts=3
  Scope1 : Scope  NumInputPorts=3
  Scope2 : Scope  NumInputPorts=3
  Zero-Order Hold : ZeroOrderHold  SampleTime=3.0517578125e-8
  Zero-Order Hold1 : ZeroOrderHold  SampleTime=3.0517578125e-8
  Data : Outport
  filter error : Outport  Port=2
  code_phase_error : Outport  Port=3
  wires:
  I_L/1 -> Rate Transition5/1
  "PRN Generator "/3(L) -> Q_L/2, I_L/2
  Q_E/1 -> Rate Transition2/1
  Q_L/1 -> Rate Transition3/1
  "PRN Generator "/2(P) -> "I_P "/2, Q_P/2
  Q_P/1 -> Rate Transition1/1
  "I_P "/1 -> Rate Transition/1
  "Carrier Loop Discriminator "/1(theta) -> Carrier Filter/1(In2), Scope1/1, Display1/1
  Rate Transition/1 -> Integrate and Dump1/1
  Rate Transition4/1 -> Integrate and Dump/1
  RT/1 -> Q_L/1, Q_P/1, Q_E/1
  Code Phase1/1 -> "PRN Generator "/3(shift)
  Product/1 -> Zero-Order Hold/1
  PRN/1 -> "PRN Generator "/1(PRN)
  Complex to Real-Imag1/2 -> Product1/2
  Input Signal/1 -> Product1/1, Product/1
  Complex to Real-Imag1/1 -> Product/2
  I_E/1 -> Rate Transition4/1
  Integrate and Dump/1 -> Scope/3, Code Loop Discriminator/1(I_E)
  Integrate and Dump5/1 -> Code Loop Discriminator/4(Q_L)
  Integrate and Dump3/1 -> Code Loop Discriminator/3(Q_E)
  "PRN Generator "/1(E) -> I_E/2, Q_E/2
  Integrate and Dump4/1 -> Display3/1, Complex to Magnitude-Angle/1
  Integrate and Dump2/1 -> Scope/1, Code Loop Discriminator/2(I_L)
  Rate Transition1/1 -> Integrate and Dump4/1
  Rate Transition3/1 -> Integrate and Dump5/1
  Rate Transition2/1 -> Integrate and Dump3/1
  Rate Transition5/1 -> Integrate and Dump2/1
  Frequency/1 -> Oscillator/2(Acq Freq)
  Product1/1 -> Zero-Order Hold1/1
  Zero-Order Hold/1 -> RT1/1
  RT1/1 -> I_E/1, I_L/1, "I_P "/1
  Integrate and Dump1/1 -> Scope/2, Display/1, Data/1, Display2/1, Complex to Magnitude-Angle1/1
  Zero-Order Hold1/1 -> RT/1
  Oscillator/1(Out1) -> Scope1/3, Complex to Real-Imag1/1
  Carrier Filter/1(Out1) -> filter error/1, Oscillator/1(phase error), Scope1/2
  Code Loop Discriminator/1(error) -> "PRN Generator "/2(error), code_phase_error/1, Scope2/1
  Complex to Magnitude-Angle/1 -> "Carrier Loop Discriminator "/2(Q_P)
  Complex to Magnitude-Angle1/1 -> "Carrier Loop Discriminator "/1(I_P)

== system Acquisition_from_autosave/Tracking Loop/Tracking Loops/Tracking Loop1/Carrier Filter ==
  In2 : Inport
  Add : Sum
  Constant : Constant  Value=0.001
  Constant1 : Constant  Value=-1
  Constant2 : Constant
  Constant3 : Constant  Value=-1
  Delay : Delay  DelayLength=1  InitialCondition=0  SampleTime=0.001
  Discrete FIR Filter : DiscreteFir  CoefSource=Input port  Coefficients=[2 1]  SampleTime=0.001
      settings: InputPortMap=u0,u1
  Discrete Filter : DiscreteFilter  NumeratorSource=Input port  DenominatorSource=Input port  SampleTime=0.001  a0EqualsOne=on
      settings: InputPortMap=u0,p1,p3
  Filter Parameters : Subsystem
  Product{,2..4} (4 alike) : Product
  Product1 : Product  Inputs=3
  Subsystem : Subsystem
  Sum : Sum  Inputs=|++
  Sum1 : Sum  Inputs=|++
  Sum3 : Sum  Inputs=|+-
  Sum4 : Sum  Inputs=+++
  Unit Delay : UnitDelay  SampleTime=0.001
  Unit Delay1 : UnitDelay  SampleTime=0.001
  Vector Concatenate : Concatenate
  Vector Concatenate1 : Concatenate
  Out1 : Outport
  wires:
  Product2/1 -> Sum/1
  Sum/1 -> Delay/1, Sum1/1
  Delay/1 -> Sum/2
  Product3/1 -> Sum1/2
  Unit Delay/1 -> Sum3/2
  Filter Parameters/1(K1) -> Product/2
  Filter Parameters/2(K2) -> Product1/2
  Constant/1 -> Product1/1
  Product1/1 -> Sum4/2
  Product/1 -> Sum4/1
  Sum4/1 -> Unit Delay1/1
  Unit Delay1/1 -> Sum4/3
  Subsystem/1("K2 ") -> Add/1, Product2/2
  Subsystem/2(K1) -> Product4/1, Add/2, Product3/1
  Sum3/1 -> Unit Delay/1, Product/1
  In2/1 -> Discrete Filter/1, Discrete FIR Filter/1, Product3/2, Product2/1
  ? -> Product1/3, Sum3/1
  Vector Concatenate/1 -> Discrete Filter/2, Discrete FIR Filter/2
  Constant1/1 -> Product4/2
  Product4/1 -> Vector Concatenate/2
  Add/1 -> Vector Concatenate/1
  Discrete Filter/1 -> Out1/1
  Constant2/1 -> Vector Concatenate1/1
  Constant3/1 -> Vector Concatenate1/2
  Vector Concatenate1/1 -> Discrete Filter/3

== system Acquisition_from_autosave/Tracking Loop/Tracking Loops/Tracking Loop1/Carrier Loop Discriminator  ==
  I_P : Inport
  Q_P : Inport  Port=2
  Constant : Constant  Value=2*pi
  Divide : Product  Inputs=/*
  Divide1 : Product  Inputs=*/
  IC : InitialCondition  Value=0
  IC1 : InitialCondition
  IC2 : InitialCondition
  atan : Trigonometry  Operator=atan
  theta : Outport
  wires:
  atan/1 -> Divide1/1
  Divide/1 -> atan/1
  I_P/1 -> IC1/1
  IC/1 -> theta/1
  Constant/1 -> Divide1/2
  Divide1/1 -> IC/1
  Q_P/1 -> IC2/1
  IC1/1 -> Divide/1
  IC2/1 -> Divide/2

== system Acquisition_from_autosave/Tracking Loop/Tracking Loops/Tracking Loop1/Code Loop Discriminator ==
  I_E : Inport
  I_L : Inport  Port=2
  Q_E : Inport  Port=3
  Q_L : Inport  Port=4
  Add : Sum
  Add1 : Sum
  Add2 : Sum  Inputs=+-
  Add3 : Sum
  Display : Display
  Divide : Product  Inputs=*/
  IC : InitialCondition  Value=0
  Math Function{,2..3,5} (4 alike) : Math  Operator=magnitude^2  RndMeth=Zero  SaturateOnIntegerOverflow=on
  Sqrt : Sqrt  SaturateOnIntegerOverflow=on
  Sqrt1 : Sqrt  SaturateOnIntegerOverflow=on
  error : Outport
  wires:
  I_L/1 -> Math Function2/1
  I_E/1 -> Math Function/1
  Q_E/1 -> Math Function3/1
  Q_L/1 -> Math Function5/1
  Math Function2/1 -> Add1/1
  Math Function5/1 -> Add1/2
  Math Function/1 -> Add/1
  Math Function3/1 -> Add/2
  Add2/1 -> Divide/1
  Add3/1 -> Divide/2
  Divide/1 -> IC/1
  IC/1 -> Display/1, error/1
  Add/1 -> Sqrt/1
  Add1/1 -> Sqrt1/1
  Sqrt/1 -> Add3/1, Add2/1
  Sqrt1/1 -> Add3/2, Add2/2

== system Acquisition_from_autosave/Tracking Loop/Tracking Loops/Tracking Loop1/Filter ==
  In2 : Inport
  Add : Sum
  Constant : Constant  Value=0.001
  Constant1 : Constant  Value=-1
  Constant2 : Constant
  Constant3 : Constant  Value=-1
  Delay : Delay  DelayLength=1  InitialCondition=0  SampleTime=0.001
  Discrete FIR Filter : DiscreteFir  CoefSource=Input port  Coefficients=[2 1]  SampleTime=0.001
      settings: InputPortMap=u0,u1
  Discrete Filter : DiscreteFilter  NumeratorSource=Input port  DenominatorSource=Input port  SampleTime=0.001  a0EqualsOne=on
      settings: InputPortMap=u0,p1,p3
  Filter Parameters : Subsystem
  Product{,2..4} (4 alike) : Product
  Product1 : Product  Inputs=3
  Subsystem : Subsystem
  Sum : Sum  Inputs=|++
  Sum1 : Sum  Inputs=|++
  Sum3 : Sum  Inputs=|+-
  Sum4 : Sum  Inputs=+++
  Unit Delay : UnitDelay  SampleTime=0.001
  Unit Delay1 : UnitDelay  SampleTime=0.001
  Vector Concatenate : Concatenate
  Vector Concatenate1 : Concatenate
  Out1 : Outport
  wires:
  Product2/1 -> Sum/1
  Sum/1 -> Delay/1, Sum1/1
  Delay/1 -> Sum/2
  Product3/1 -> Sum1/2
  Unit Delay/1 -> Sum3/2
  Filter Parameters/1(K1) -> Product/2
  Filter Parameters/2(K2) -> Product1/2
  Constant/1 -> Product1/1
  Product1/1 -> Sum4/2
  Product/1 -> Sum4/1
  Sum4/1 -> Unit Delay1/1
  Unit Delay1/1 -> Sum4/3
  Subsystem/1("K2 ") -> Add/1, Product2/2
  Subsystem/2(K1) -> Product4/1, Add/2, Product3/1
  Sum3/1 -> Unit Delay/1, Product/1
  In2/1 -> Discrete Filter/1, Discrete FIR Filter/1, Product3/2, Product2/1
  ? -> Product1/3, Sum3/1
  Vector Concatenate/1 -> Discrete Filter/2, Discrete FIR Filter/2
  Constant1/1 -> Product4/2
  Product4/1 -> Vector Concatenate/2
  Add/1 -> Vector Concatenate/1
  Discrete Filter/1 -> Out1/1
  Constant2/1 -> Vector Concatenate1/1
  Constant3/1 -> Vector Concatenate1/2
  Vector Concatenate1/1 -> Discrete Filter/3

== system Acquisition_from_autosave/Tracking Loop/Tracking Loops/Tracking Loop1/Oscillator ==
  phase error : Inport
  Acq Freq : Inport  Port=2
  2*pi2 : Constant  Value=2*pi
  2^N2 : Constant  Value=2^16
  Add : Sum
  Counter Free-Running : simulink/Sources/Counter Free-Running  NumBits=15  tsamp=1/32768000
  Divide1 : Product  Inputs=*/
  Divide10 : Product
  Divide8 : Product  Inputs=*/*
  Divide9 : Product  Inputs=***
  Fs2 : Constant  Value=32768000
  IC : InitialCondition  Value=9207000
  MATLAB Function2 : MATLAB Function  TreatAsAtomicUnit=on
  Math Function : Math  Operator=mod  SaturateOnIntegerOverflow=on
  Pulse Generator1 : DiscretePulseGenerator  PulseType=Time based  Period=0.005  PulseWidth=50
  RT2 : RateTransition
  Real-Imag to Complex2 : RealImagToComplex
  Resettable Delay : Delay  DelayLength=1  ExternalReset=Rising  SampleTime=0.001
      settings: InputPortMap=u0,r5
  Sum2 : Sum  Inputs=-+|
  Out1 : Outport
  wires:
  2*pi2/1 -> Divide9/3, Divide10/1
  Sum2/1 -> Divide9/1
  Divide8/1 -> Sum2/2
  2^N2/1 -> Divide10/2, Divide1/2, Divide9/2
  Fs2/1 -> Divide8/2
  Divide10/1 -> Math Function/2
  phase error/1 -> Sum2/1
  Acq Freq/1 -> Divide8/1
  Pulse Generator1/1 -> RT2/1
  MATLAB Function2/1(I) -> Real-Imag to Complex2/1
  MATLAB Function2/2(Q) -> Real-Imag to Complex2/2
  Divide1/1 -> IC/1
  IC/1 -> MATLAB Function2/1(u)
  Resettable Delay/1 -> Add/1
  Math Function/1 -> Resettable Delay/1, Divide1/1
  Add/1 -> Math Function/1
  Divide9/1 -> Add/2
  Real-Imag to Complex2/1 -> Out1/1
  Counter Free-Running/1 -> Divide8/3

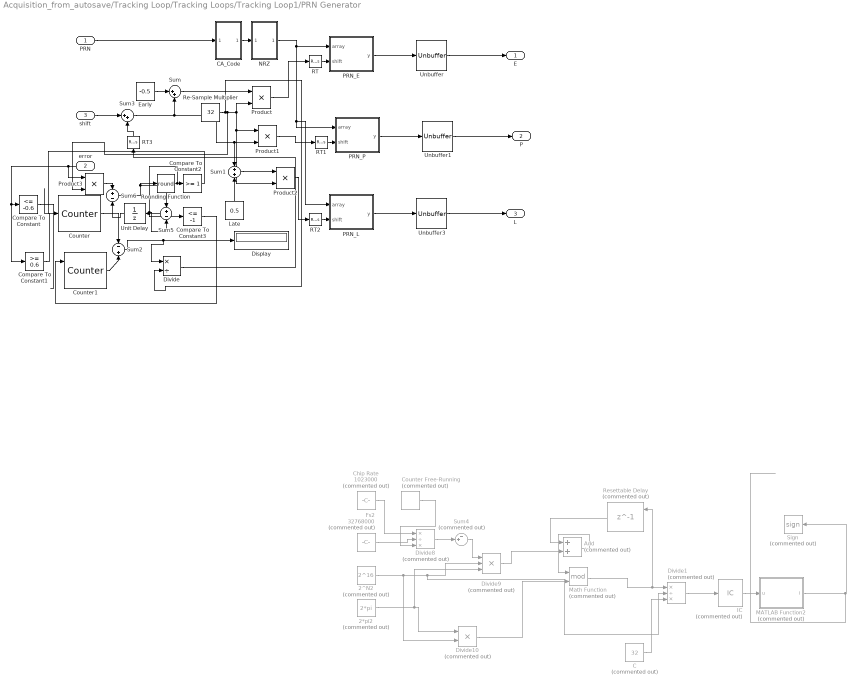
== system Acquisition_from_autosave/Tracking Loop/Tracking Loops/Tracking Loop1/PRN Generator  ==
  PRN : Inport
  error : Inport  Port=2  SampleTime=0.001
  shift : Inport  Port=3
  2*pi2 : Constant  Commented=on  Value=2*pi
  2^N2 : Constant  Commented=on  Value=2^16
  Add : Sum  Commented=on
  C : Constant  Commented=on  Value=32
  "CA_Code " : Subsystem
  Chip Rate : Constant  Commented=on  Value=1023000
  Compare To Constant : simulink/Logic and Bit Operations/Compare To Constant  relop=<=  const=-0.6  OutDataTypeStr=boolean
  Compare To Constant1 : simulink/Logic and Bit Operations/Compare To Constant  relop=>=  const=0.6  OutDataTypeStr=boolean
  Compare To Constant2 : simulink/Logic and Bit Operations/Compare To Constant  relop=>=  const=1  OutDataTypeStr=uint8
  Compare To Constant3 : simulink/Logic and Bit Operations/Compare To Constant  relop=<=  const=-1  OutDataTypeStr=uint8
  Counter : dspswit3/Counter  Direction=Up  CountEvent=Non-zero sample  CounterSize=User defined  MaxCount=255  InitialCount=0  Output=Count  HitValue=32  ResetInput=off  SamplesPerFrame=1  Ts=1  CntDtype=double  HitDtype=Logical
  Counter Free-Running : simulink/Sources/Counter Free-Running  Commented=on  NumBits=15  tsamp=1/32768000
  Counter1 : dspswit3/Counter  Direction=Up  CountEvent=Non-zero sample  CounterSize=User defined  MaxCount=255  InitialCount=0  Output=Count  HitValue=32  ResetInput=on  SamplesPerFrame=1  Ts=1  CntDtype=double  HitDtype=Logical
  Display : Display
  Divide : Product  Inputs=*/
  Divide1 : Product  Commented=on  Inputs=*/*
  Divide10 : Product  Commented=on
  Divide8 : Product  Commented=on  Inputs=*/*
  Divide9 : Product  Commented=on  Inputs=***
  Early : Constant  Value=-0.5
  Fs2 : Constant  Commented=on  Value=32768000
  IC : InitialCondition  Commented=on  Value=1023000
  Late : Constant  Value=0.5
  MATLAB Function2 : MATLAB Function  Commented=on  TreatAsAtomicUnit=on
  Math Function : Math  Commented=on  Operator=mod  SaturateOnIntegerOverflow=on
  NRZ : Subsystem
  PRN_E : MATLAB Function  TreatAsAtomicUnit=on  SystemSampleTime=0.001
  PRN_L : MATLAB Function  TreatAsAtomicUnit=on  SystemSampleTime=0.001
  PRN_P : MATLAB Function  TreatAsAtomicUnit=on  SystemSampleTime=0.001
  Product{,1..3} (4 alike) : Product
  RT : RateTransition  OutPortSampleTime=0.001
  RT1 : RateTransition  OutPortSampleTime=0.001
  RT2 : RateTransition  OutPortSampleTime=0.001
  RT3 : RateTransition
  Re-Sample Multiplier : Constant  Value=32
  Resettable Delay : Delay  Commented=on  DelayLength=1  ExternalReset=Rising  SampleTime=0.001
      settings: InputPortMap=u0,r5
  Rounding Function : Rounding  Operator=round
  Sign : Signum  Commented=on
  Sum : Sum  Inputs=|++
  Sum1 : Sum
  Sum2 : Sum  Inputs=-+
  Sum3 : Sum  Inputs=|++
  Sum4 : Sum  Commented=on  Inputs=-+|
  Sum5 : Sum  Inputs=+-
  Sum6 : Sum  Inputs=+-
  Unbuffer : Unbuffer
  Unbuffer1 : Unbuffer
  Unbuffer3 : Unbuffer
  Unit Delay : UnitDelay  SampleTime=0.001
  E : Outport
  P : Outport  Port=2
  L : Outport  Port=3
  wires:
  Product/1 -> RT/1
  PRN_E/1(y) -> Unbuffer/1
  Product2/1 -> RT2/1
  PRN_L/1(y) -> Unbuffer3/1
  Re-Sample Multiplier/1 -> Divide/2, Product3/2, Product1/1, Product2/2, Product/2
  PRN/1 -> "CA_Code "/1(In1)
  Unbuffer1/1 -> P/1
  Unbuffer3/1 -> L/1
  Early/1 -> Sum/1
  Sum/1 -> Product/1
  Sum3/1 -> Product1/2, Sum1/1, Sum/2
  Sum1/1 -> Product2/1
  PRN_P/1(y) -> Unbuffer1/1
  error/1 -> Product3/1, Compare To Constant1/1, Compare To Constant/1
  Counter/1 -> Sum2/1
  Counter1/1 -> Sum2/2
  Sum2/1 -> Divide/1, Display/1
  shift/1 -> Sum3/1
  RT/1 -> PRN_E/2(shift)
  RT1/1 -> PRN_P/2(shift)
  RT2/1 -> PRN_L/2(shift)
  Late/1 -> Sum1/2
  "CA_Code "/1(Out1) -> NRZ/1(In1)
  Unbuffer/1 -> E/1
  NRZ/1(Out1) -> PRN_E/1(array), PRN_L/1(array), PRN_P/1(array)
  Product1/1 -> RT1/1
  RT3/1 -> Sum3/2
  Compare To Constant1/1 -> ?
  Compare To Constant/1 -> ?
  MATLAB Function2/1(I) -> Sign/1
  Divide8/1 -> Sum4/2
  C/1 -> Divide1/3
  2^N2/1 -> Divide10/2, Divide1/2, Divide9/2
  Fs2/1 -> Divide8/2
  2*pi2/1 -> Divide9/3, Divide10/1
  Sum4/1 -> Divide9/1
  IC/1 -> MATLAB Function2/1(u)
  Divide10/1 -> Math Function/2
  Chip Rate/1 -> Divide8/1
  Resettable Delay/1 -> Add/1
  Divide1/1 -> IC/1
  Divide9/1 -> Add/2
  Counter Free-Running/1 -> Divide8/3
  Add/1 -> Math Function/1
  Math Function/1 -> Resettable Delay/1, Divide1/1
  Compare To Constant2/1 -> Counter/1
  Compare To Constant3/1 -> Counter1/1
  Divide/1 -> RT3/1
  Rounding Function/1 -> Sum5/2, Compare To Constant3/1, Compare To Constant2/1
  Product3/1 -> Sum6/1
  Sum5/1 -> Unit Delay/1
  Sum6/1 -> Sum5/1, Rounding Function/1
  Unit Delay/1 -> Sum6/2

== system Acquisition_from_autosave/Tracking Loop/Tracking Loops/Tracking Loop2/Carrier Filter ==
  In2 : Inport
  Add : Sum
  Constant : Constant  Value=0.001
  Constant1 : Constant  Value=-1
  Constant2 : Constant
  Constant3 : Constant  Value=-1
  Delay : Delay  DelayLength=1  InitialCondition=0  SampleTime=0.001
  Discrete FIR Filter : DiscreteFir  CoefSource=Input port  Coefficients=[2 1]  SampleTime=0.001
      settings: InputPortMap=u0,u1
  Discrete Filter : DiscreteFilter  NumeratorSource=Input port  DenominatorSource=Input port  SampleTime=0.001  a0EqualsOne=on
      settings: InputPortMap=u0,p1,p3
  Filter Parameters : Subsystem
  Product{,2..4} (4 alike) : Product
  Product1 : Product  Inputs=3
  Subsystem : Subsystem
  Sum : Sum  Inputs=|++
  Sum1 : Sum  Inputs=|++
  Sum3 : Sum  Inputs=|+-
  Sum4 : Sum  Inputs=+++
  Unit Delay : UnitDelay  SampleTime=0.001
  Unit Delay1 : UnitDelay  SampleTime=0.001
  Vector Concatenate : Concatenate
  Vector Concatenate1 : Concatenate
  Out1 : Outport
  wires:
  Product2/1 -> Sum/1
  Sum/1 -> Delay/1, Sum1/1
  Delay/1 -> Sum/2
  Product3/1 -> Sum1/2
  Unit Delay/1 -> Sum3/2
  Filter Parameters/1(K1) -> Product/2
  Filter Parameters/2(K2) -> Product1/2
  Constant/1 -> Product1/1
  Product1/1 -> Sum4/2
  Product/1 -> Sum4/1
  Sum4/1 -> Unit Delay1/1
  Unit Delay1/1 -> Sum4/3
  Subsystem/1("K2 ") -> Add/1, Product2/2
  Subsystem/2(K1) -> Product4/1, Add/2, Product3/1
  Sum3/1 -> Unit Delay/1, Product/1
  In2/1 -> Discrete Filter/1, Discrete FIR Filter/1, Product3/2, Product2/1
  ? -> Product1/3, Sum3/1
  Vector Concatenate/1 -> Discrete Filter/2, Discrete FIR Filter/2
  Constant1/1 -> Product4/2
  Product4/1 -> Vector Concatenate/2
  Add/1 -> Vector Concatenate/1
  Discrete Filter/1 -> Out1/1
  Constant2/1 -> Vector Concatenate1/1
  Constant3/1 -> Vector Concatenate1/2
  Vector Concatenate1/1 -> Discrete Filter/3

== system Acquisition_from_autosave/Tracking Loop/Tracking Loops/Tracking Loop2/Carrier Loop Discriminator  ==
  I_P : Inport
  Q_P : Inport  Port=2
  Constant : Constant  Value=2*pi
  Divide : Product  Inputs=/*
  Divide1 : Product  Inputs=*/
  IC : InitialCondition  Value=0
  IC1 : InitialCondition
  IC2 : InitialCondition
  atan : Trigonometry  Operator=atan
  theta : Outport
  wires:
  atan/1 -> Divide1/1
  Divide/1 -> atan/1
  I_P/1 -> IC1/1
  IC/1 -> theta/1
  Constant/1 -> Divide1/2
  Divide1/1 -> IC/1
  Q_P/1 -> IC2/1
  IC1/1 -> Divide/1
  IC2/1 -> Divide/2

== system Acquisition_from_autosave/Tracking Loop/Tracking Loops/Tracking Loop2/Code Filter ==
  In1 : Inport  SampleTime=0.001
  Add : Sum
  BW : Constant  Value=25
  Coeffiecients : Subsystem
  Constant : Constant  Value=2*pi
  Delay : Delay  DelayLength=1  InitialCondition=0  SampleTime=0.001
  Delay1 : Delay  DelayLength=1  InitialCondition=0  SampleTime=0.001
  Display : Display
  Display1 : Display
  Divide : Product  Inputs=*/
  Divide1 : Product  Inputs=**
  Divide2 : Product  Inputs=**
  Subtract : Sum  Inputs=-++
  ts : Constant  Value=0.001
  zeta : Constant  Value=0.7
  Out1 : Outport
  wires:
  Constant/1 -> Divide/2
  Divide/1 -> Delay/1, Divide2/1
  BW/1 -> Coeffiecients/1(BW)
  zeta/1 -> Coeffiecients/2(Zeta)
  ts/1 -> Coeffiecients/3(ts)
  Coeffiecients/1(C1) -> Add/1, Divide1/2
  Delay/1 -> Divide1/1
  Coeffiecients/2(C2) -> Add/2
  Add/1 -> Divide2/2
  Divide1/1 -> Subtract/1
  Divide2/1 -> Subtract/2
  Subtract/1 -> Out1/1, Delay1/1
  Delay1/1 -> Subtract/3
  In1/1 -> Divide/1

== system Acquisition_from_autosave/Tracking Loop/Tracking Loops/Tracking Loop2/Code Loop Discriminator ==
  I_E : Inport
  I_L : Inport  Port=2
  Q_E : Inport  Port=3
  Q_L : Inport  Port=4
  Add : Sum
  Add1 : Sum
  Add2 : Sum  Inputs=+-
  Add3 : Sum
  Display : Display
  Divide : Product  Inputs=*/
  IC : InitialCondition  Value=0
  Math Function{,2..3,5} (4 alike) : Math  Operator=magnitude^2  RndMeth=Zero  SaturateOnIntegerOverflow=on
  Sqrt : Sqrt  SaturateOnIntegerOverflow=on
  Sqrt1 : Sqrt  SaturateOnIntegerOverflow=on
  error : Outport
  wires:
  I_L/1 -> Math Function2/1
  I_E/1 -> Math Function/1
  Q_E/1 -> Math Function3/1
  Q_L/1 -> Math Function5/1
  Math Function2/1 -> Add1/1
  Math Function5/1 -> Add1/2
  Math Function/1 -> Add/1
  Math Function3/1 -> Add/2
  Add2/1 -> Divide/1
  Add3/1 -> Divide/2
  Divide/1 -> IC/1
  IC/1 -> Display/1, error/1
  Add/1 -> Sqrt/1
  Add1/1 -> Sqrt1/1
  Sqrt/1 -> Add3/1, Add2/1
  Sqrt1/1 -> Add3/2, Add2/2

== system Acquisition_from_autosave/Tracking Loop/Tracking Loops/Tracking Loop2/Controlled Carrier Generator ==
  Freq ACQ : Inport
  Phase Error : Inport  Port=2
  Freq Error : Inport  Port=3
  Clock : Clock  Commented=on
  Clock1 : Clock
  Discrete Derivative : simulink/Discrete/Discrete Derivative  gainval=1.0  ICPrevScaledInput=0.0  OutMin=[]  OutMax=[]  OutDataType=fixdt(1, 16)  OutScaling=2^-10  DoSatur=off
  Display : Display
  MATLAB Function : MATLAB Function  TreatAsAtomicUnit=on
  MATLAB Function1 : MATLAB Function  Commented=on  TreatAsAtomicUnit=on
  Sum : Sum  Inputs=++|
  "wave " : Outport
  wires:
  Clock/1 -> MATLAB Function1/2(timer)
  Freq Error/1 -> Sum/1
  Freq ACQ/1 -> Sum/2
  Sum/1 -> MATLAB Function/2(freq)
  Clock1/1 -> MATLAB Function/1(time)
  Phase Error/1 -> Discrete Derivative/1, MATLAB Function/3(phase)
  MATLAB Function/1(wave) -> "wave "/1
  Discrete Derivative/1 -> Display/1

== system Acquisition_from_autosave/Tracking Loop/Tracking Loops/Tracking Loop2/Oscillator ==
  phase error : Inport
  Acq Freq : Inport  Port=2
  2*pi2 : Constant  Value=2*pi
  2^N2 : Constant  Value=2^16
  Add : Sum
  Counter Free-Running : simulink/Sources/Counter Free-Running  NumBits=15  tsamp=1/32768000
  Divide1 : Product  Inputs=*/
  Divide10 : Product
  Divide8 : Product  Inputs=*/*
  Divide9 : Product  Inputs=***
  Fs2 : Constant  Value=32768000
  IC : InitialCondition  Value=9207000
  MATLAB Function2 : MATLAB Function  TreatAsAtomicUnit=on
  Math Function : Math  Operator=mod  SaturateOnIntegerOverflow=on
  Pulse Generator1 : DiscretePulseGenerator  PulseType=Time based  Period=0.005  PulseWidth=50
  RT2 : RateTransition
  Real-Imag to Complex2 : RealImagToComplex
  Resettable Delay : Delay  DelayLength=1  ExternalReset=Rising  SampleTime=0.001
      settings: InputPortMap=u0,r5
  Sum2 : Sum  Inputs=-+|
  Out1 : Outport
  wires:
  2*pi2/1 -> Divide9/3, Divide10/1
  Sum2/1 -> Divide9/1
  Divide8/1 -> Sum2/2
  2^N2/1 -> Divide10/2, Divide1/2, Divide9/2
  Fs2/1 -> Divide8/2
  Divide10/1 -> Math Function/2
  phase error/1 -> Sum2/1
  Acq Freq/1 -> Divide8/1
  Pulse Generator1/1 -> RT2/1
  MATLAB Function2/1(I) -> Real-Imag to Complex2/1
  MATLAB Function2/2(Q) -> Real-Imag to Complex2/2
  Divide1/1 -> IC/1
  IC/1 -> MATLAB Function2/1(u)
  Resettable Delay/1 -> Add/1
  Math Function/1 -> Resettable Delay/1, Divide1/1
  Add/1 -> Math Function/1
  Divide9/1 -> Add/2
  Real-Imag to Complex2/1 -> Out1/1
  Counter Free-Running/1 -> Divide8/3
